simulink model "sampleModel1669"  (R2023a)
settings: Solver=VariableStepAuto  StartTime=0.0  StopTime=10.0  RelTol=1e-3
libraries: hdlsllib x4
settings Model: Creator=user1  LastModifiedBy=user1

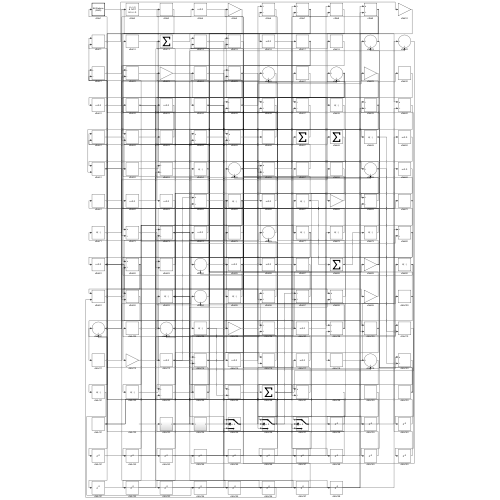
[thumbnail: Simulink's stored preview of the top-level diagram]
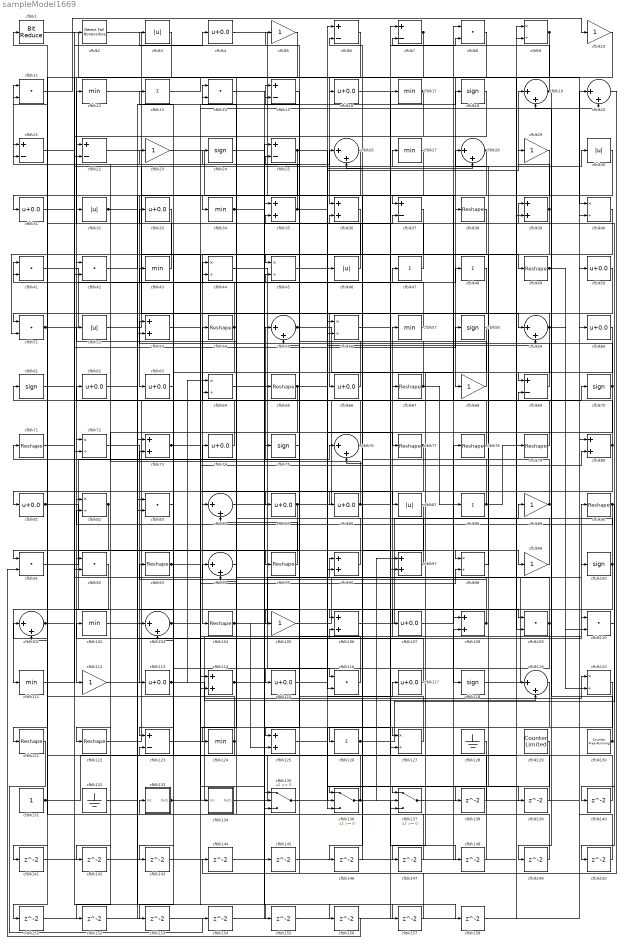
== system sampleModel1669 ==
  cfblk1 : hdlsllib/Logic and Bit Operations/Bit Reduce  mode=AND
  cfblk{5,10,23,29,68,89,99,105,112} (9 alike) : Gain
  cfblk{18,24,58,61,70,75,100,118} (8 alike) : Signum
  cfblk{19..20,26,28,55,59,76,84,94,101,103,119} (12 alike) : Sum  Inputs=|++
  cfblk{12,17,27,34,43,57,102,111,124} (9 alike) : MinMax
  cfblk{38,49,54,65,67,71,77..79,90,93,95,104,121..122} (15 alike) : Reshape
  cfblk{35..36,39,53,73,80,96..97,106,108,114,125} (12 alike) : Sum
  cfblk{4,16,31,33,50,60,62..63,66,74,81,85..86,107,113,115,117} (17 alike) : Bias  Bias=0.0  SaturateOnIntegerOverflow=off
  cfblk{8,11,14,41..42,51,83,91..92,109..110,116} (12 alike) : DotProduct  OutDataTypeStr=Inherit: Inherit via internal rule
  cfblk{9,40,44..45,56,64,72,82,98,120,127} (11 alike) : Product  Inputs=*/  RndMeth=Zero  SaturateOnIntegerOverflow=on
  cfblk{6..7,15,21..22,25,37,69,123} (9 alike) : Sum  Inputs=+-
  cfblk{13,47..48,88,126} (5 alike) : Sum  Inputs=+
  cfblk128 : Ground
  cfblk129 : hdlsllib/Sources/Counter Limited  uplimit=7  tsamp=-1
  cfblk130 : hdlsllib/Sources/Counter Free-Running  NumBits=16  tsamp=-1
  cfblk131 : Constant  SampleTime=-1
  cfblk132 : Ground
  cfblk133 : Subsystem
      settings: LibrarySourceBlock=|
      | hdlsllib/Ports &
      | Subsystems/Subsystem
  cfblk134 : Subsystem
      settings: LibrarySourceBlock=|
      | hdlsllib/Ports &
      | Subsystems/Subsystem
  cfblk135 : Switch  SaturateOnIntegerOverflow=off  InputSameDT=off
  cfblk136 : Switch  SaturateOnIntegerOverflow=off  InputSameDT=off
  cfblk137 : Switch  SaturateOnIntegerOverflow=off  InputSameDT=off
  cfblk{138..158} (21 alike) : Delay  SampleTime=1
  cfblk2 : hdlsllib/Logic and Bit Operations/Detect Fall Nonpositive  vinit=0  OutDataTypeStr=boolean
  cfblk{3,30,32,46,52,87} (6 alike) : Abs  SaturateOnIntegerOverflow=off
  wires:
  cfblk104/1 -> cfblk96/1, cfblk125/2
  cfblk38/1 -> cfblk104/1
  cfblk7/1 -> cfblk112/1, cfblk92/2
  cfblk35/1 -> cfblk11/1, cfblk29/1
  cfblk122/1 -> cfblk90/1
  cfblk67/1 -> cfblk88/1, cfblk6/2
  cfblk84/1 -> cfblk99/1
  cfblk17/1 -> cfblk72/1, cfblk42/2
  cfblk133/1(Out1) -> cfblk120/1, cfblk110/1
  cfblk68/1 -> cfblk41/1
  cfblk2/1 -> cfblk34/1
  cfblk126/1 -> cfblk39/1, cfblk8/2
  cfblk43/1 -> cfblk12/1
  cfblk105/1 -> cfblk100/1
  cfblk128/1 -> cfblk133/1(In1)
  cfblk28/1 -> cfblk31/1, cfblk97/2, cfblk146/1
  cfblk10/1 -> cfblk84/1
  cfblk44/1 -> cfblk116/1
  cfblk118/1 -> cfblk50/1
  cfblk12/1 -> cfblk59/1
  cfblk30/1 -> cfblk42/1
  cfblk106/1 -> cfblk89/1
  cfblk91/1 -> cfblk55/1
  cfblk123/1 -> cfblk57/1
  cfblk26/1 -> cfblk63/1
  cfblk87/1 -> cfblk136/1
  cfblk50/1 -> cfblk105/1
  cfblk86/1 -> cfblk62/1, cfblk98/1
  cfblk11/1 -> cfblk10/1
  cfblk131/1 -> cfblk21/1, cfblk73/1, cfblk9/2
  cfblk19/1 -> cfblk69/1, cfblk7/2
  cfblk76/1 -> cfblk54/1
  cfblk109/1 -> cfblk71/1, cfblk153/1
  cfblk25/1 -> cfblk116/2, cfblk83/2
  cfblk52/1 -> cfblk27/1
  cfblk6/1 -> cfblk36/1
  cfblk18/1 -> cfblk85/1
  cfblk61/1 -> cfblk4/1
  cfblk33/1 -> cfblk72/2
  cfblk45/1 -> cfblk6/1
  cfblk100/1 -> cfblk126/1, cfblk52/1
  cfblk117/1 -> cfblk102/1
  cfblk64/1 -> cfblk87/1
  cfblk8/1 -> cfblk68/1
  cfblk89/1 -> cfblk67/1, cfblk19/2
  cfblk22/1 -> cfblk45/1
  cfblk41/1 -> cfblk45/2
  cfblk101/1 -> cfblk30/1, cfblk58/1
  cfblk137/1 -> cfblk60/1
  cfblk129/1 -> cfblk136/2
  cfblk4/1 -> cfblk37/1
  cfblk48/1 -> cfblk66/1
  cfblk23/1 -> cfblk108/1
  cfblk113/1 -> cfblk119/2, cfblk64/1, cfblk80/2
  cfblk62/1 -> cfblk44/1
  cfblk107/1 -> cfblk78/1
  cfblk97/1 -> cfblk74/1
  cfblk29/1 -> cfblk95/1
  cfblk83/1 -> cfblk23/1
  cfblk51/1 -> cfblk7/1, cfblk107/1
  cfblk59/1 -> cfblk51/1, cfblk120/2, cfblk103/2
  cfblk65/1 -> cfblk122/1, cfblk77/1, cfblk28/2, cfblk82/1
  cfblk94/1 -> cfblk44/2
  cfblk46/1 -> cfblk21/2
  cfblk120/1 -> cfblk136/3
  cfblk70/1 -> cfblk53/1, cfblk152/1
  cfblk78/1 -> cfblk14/1
  cfblk53/1 -> cfblk18/1
  cfblk95/1 -> cfblk84/2
  cfblk37/1 -> cfblk51/2
  cfblk77/1 -> cfblk94/2, cfblk142/1
  cfblk27/1 -> cfblk106/1
  cfblk92/1 -> cfblk111/1
  cfblk135/1 -> cfblk117/1
  cfblk71/1 -> cfblk70/1
  cfblk47/1 -> cfblk14/2
  cfblk15/1 -> cfblk125/1
  cfblk66/1 -> cfblk3/1
  cfblk112/1 -> cfblk20/1
  cfblk60/1 -> cfblk115/1
  cfblk75/1 -> cfblk35/2
  cfblk81/1 -> cfblk114/1, cfblk137/3, cfblk157/1
  cfblk99/1 -> cfblk65/1
  cfblk96/1 -> cfblk33/1
  cfblk134/1(Out1) -> cfblk17/1
  cfblk34/1 -> cfblk49/1, cfblk109/1
  cfblk57/1 -> cfblk43/1
  cfblk88/1 -> cfblk32/1, cfblk79/1
  cfblk55/1 -> cfblk118/1, cfblk59/2
  cfblk103/1 -> cfblk134/1(In1), cfblk98/2
  cfblk1/1 -> cfblk40/1
  cfblk3/1 -> cfblk91/1
  cfblk79/1 -> cfblk61/1
  cfblk13/1 -> cfblk16/1
  cfblk16/1 -> cfblk38/1
  cfblk5/1 -> cfblk81/1
  cfblk9/1 -> cfblk124/1, cfblk109/2
  cfblk21/1 -> cfblk2/1
  cfblk115/1 -> cfblk46/1
  cfblk130/1 -> cfblk69/2, cfblk36/2
  cfblk85/1 -> cfblk8/1, cfblk151/1
  cfblk90/1 -> cfblk82/2, cfblk140/1
  cfblk116/1 -> cfblk15/1
  cfblk56/1 -> cfblk48/1
  cfblk72/1 -> cfblk113/1
  cfblk108/1 -> cfblk93/1, cfblk26/2
  cfblk36/1 -> cfblk114/2
  cfblk127/1 -> cfblk75/1
  cfblk42/1 -> cfblk15/2
  cfblk114/1 -> cfblk26/1, cfblk37/2
  cfblk73/1 -> cfblk47/1, cfblk127/2, cfblk86/1
  cfblk111/1 -> cfblk94/1
  cfblk49/1 -> cfblk110/2, cfblk149/1
  cfblk39/1 -> cfblk19/1, cfblk123/1, cfblk138/1
  cfblk102/1 -> cfblk76/1
  cfblk74/1 -> cfblk22/1
  cfblk119/1 -> cfblk127/1
  cfblk40/1 -> cfblk56/2
  cfblk69/1 -> cfblk25/2
  cfblk32/1 -> cfblk96/2, cfblk156/1
  cfblk124/1 -> cfblk24/1, cfblk101/2, cfblk123/2
  cfblk136/1 -> cfblk101/1, cfblk97/1, cfblk73/2, cfblk148/1
  cfblk98/1 -> cfblk28/1
  cfblk54/1 -> cfblk103/1, cfblk13/1
  cfblk93/1 -> cfblk135/2, cfblk20/2, cfblk155/1
  cfblk82/1 -> cfblk92/1, cfblk141/1
  cfblk80/1 -> cfblk137/1, cfblk41/2, cfblk121/1
  cfblk31/1 -> cfblk22/2
  cfblk132/1 -> cfblk106/2
  cfblk138/1 -> cfblk56/1
  cfblk125/1 -> cfblk139/1
  cfblk139/1 -> cfblk25/1
  cfblk140/1 -> cfblk11/2
  cfblk141/1 -> cfblk83/1
  cfblk142/1 -> cfblk35/1
  cfblk63/1 -> cfblk143/1
  cfblk143/1 -> cfblk108/2
  cfblk20/1 -> cfblk144/1
  cfblk144/1 -> cfblk119/1
  cfblk14/1 -> cfblk145/1
  cfblk145/1 -> cfblk55/2
  cfblk146/1 -> cfblk76/2
  cfblk58/1 -> cfblk147/1
  cfblk147/1 -> cfblk1/1
  cfblk148/1 -> cfblk64/2
  cfblk149/1 -> cfblk135/1
  cfblk110/1 -> cfblk150/1
  cfblk150/1 -> cfblk80/1
  cfblk151/1 -> cfblk53/2
  cfblk152/1 -> cfblk137/2
  cfblk153/1 -> cfblk135/3
  cfblk121/1 -> cfblk154/1
  cfblk154/1 -> cfblk39/2
  cfblk155/1 -> cfblk40/2
  cfblk156/1 -> cfblk91/2
  cfblk157/1 -> cfblk5/1
  cfblk24/1 -> cfblk158/1
  cfblk158/1 -> cfblk9/1

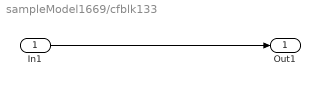
== system sampleModel1669/cfblk133 ==
  In1 : Inport
  Out1 : Outport
  wires:
  In1/1 -> Out1/1

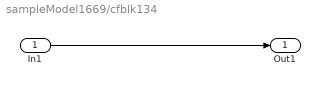
== system sampleModel1669/cfblk134 ==
  In1 : Inport
  Out1 : Outport
  wires:
  In1/1 -> Out1/1
